simulink model "bhxxx_SL"  (R2016b)
settings: Solver=ode15s  StartTime=0.0  StopTime=60  FixedStep=0.001  RelTol=1e-5  EnableMultiTasking=on
undefined symbols (not defined in the file): b1_damp, b2_damp, b3_damp, b4_damp, g, L1x, L1y, L1z, L2x, L2y, L2z, L3x, L3y, L3z, mass1, mass2, mass3, mass4, Rturn, theta1_0, theta1_dot_0, theta2_0, theta2_dot_0, theta3_0, theta3_dot_0, theta4_0, theta4_dot_0
libraries: simulink x9, discretizing x4, simulink_extras x2
(part 2 of 2)

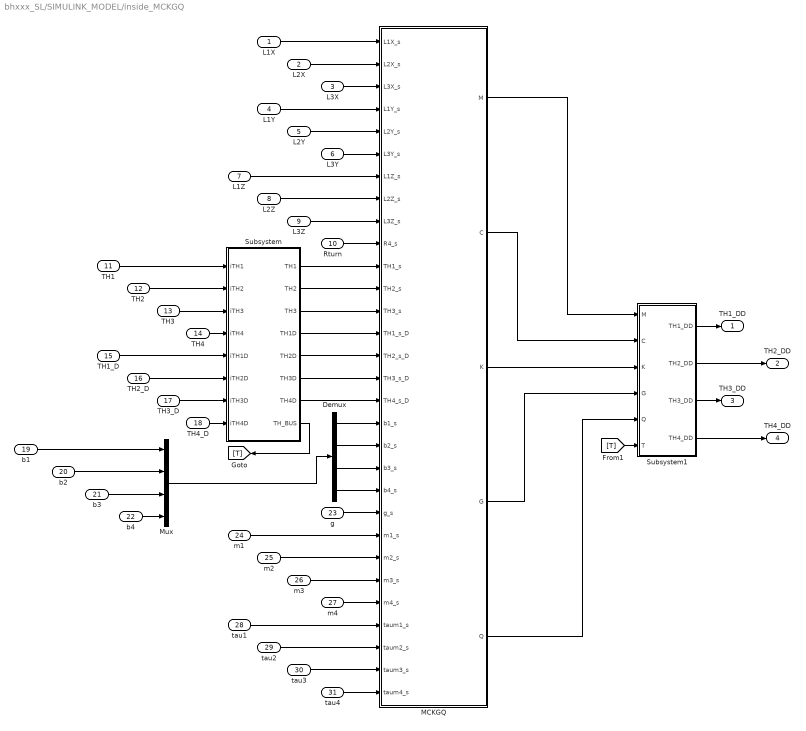
== system bhxxx_SL/SIMULINK_MODEL/inside_MCKGQ ==
  L1X : Inport
  L2X : Inport  Port=2
  L3X : Inport  Port=3
  L1Y : Inport  Port=4
  L2Y : Inport  Port=5
  L3Y : Inport  Port=6
  L1Z : Inport  Port=7
  L2Z : Inport  Port=8
  L3Z : Inport  Port=9
  Rturn : Inport  Port=10
  TH1 : Inport  Port=11
  TH2 : Inport  Port=12
  TH3 : Inport  Port=13
  TH4 : Inport  Port=14
  TH1_D : Inport  Port=15
  TH2_D : Inport  Port=16
  TH3_D : Inport  Port=17
  TH4_D : Inport  Port=18
  b1 : Inport  Port=19
  b2 : Inport  Port=20
  b3 : Inport  Port=21
  b4 : Inport  Port=22
  g : Inport  Port=23
  m1 : Inport  Port=24
  m2 : Inport  Port=25
  m3 : Inport  Port=26
  m4 : Inport  Port=27
  tau1 : Inport  Port=28
  tau2 : Inport  Port=29
  tau3 : Inport  Port=30
  tau4 : Inport  Port=31
  Demux : Demux
  MCKGQ : MATLAB Function  TreatAsAtomicUnit=on
  Mux : Mux
  Subsystem : Subsystem
  Subsystem1 : Subsystem
  TH1_DD : Outport
  TH2_DD : Outport  Port=2
  TH3_DD : Outport  Port=3
  TH4_DD : Outport  Port=4
  wires:
  m2/1 -> MCKGQ/24(m2_s)
  m3/1 -> MCKGQ/25(m3_s)
  m4/1 -> MCKGQ/26(m4_s)
  tau1/1 -> MCKGQ/27(taum1_s)
  g/1 -> MCKGQ/22(g_s)
  m1/1 -> MCKGQ/23(m1_s)
  TH1_D/1 -> Subsystem/5(iTH1D)
  b1/1 -> Mux/1
  b2/1 -> Mux/2
  TH3/1 -> Subsystem/3(iTH3)
  b3/1 -> Mux/3
  TH4_D/1 -> Subsystem/8(iTH4D)
  TH2_D/1 -> Subsystem/6(iTH2D)
  TH3_D/1 -> Subsystem/7(iTH3D)
  b4/1 -> Mux/4
  tau2/1 -> MCKGQ/28(taum2_s)
  tau3/1 -> MCKGQ/29(taum3_s)
  tau4/1 -> MCKGQ/30(taum4_s)
  L2X/1 -> MCKGQ/2(L2X_s)
  L3X/1 -> MCKGQ/3(L3X_s)
  L2Y/1 -> MCKGQ/5(L2Y_s)
  L3Y/1 -> MCKGQ/6(L3Y_s)
  L1Y/1 -> MCKGQ/4(L1Y_s)
  L2Z/1 -> MCKGQ/8(L2Z_s)
  L3Z/1 -> MCKGQ/9(L3Z_s)
  L1Z/1 -> MCKGQ/7(L1Z_s)
  TH1/1 -> Subsystem/1(iTH1)
  Rturn/1 -> MCKGQ/10(R4_s)
  TH2/1 -> Subsystem/2(iTH2)
  L1X/1 -> MCKGQ/1(L1X_s)
  Subsystem/8(TH_BUS) -> [T]
  Subsystem/7(TH4D) -> MCKGQ/17(TH4_s_D)
  Subsystem/6(TH3D) -> MCKGQ/16(TH3_s_D)
  Subsystem/5(TH2D) -> MCKGQ/15(TH2_s_D)
  Subsystem/4(TH1D) -> MCKGQ/14(TH1_s_D)
  Subsystem/3(TH3) -> MCKGQ/13(TH3_s)
  Subsystem/2(TH2) -> MCKGQ/12(TH2_s)
  Subsystem/1(TH1) -> MCKGQ/11(TH1_s)
  TH4/1 -> Subsystem/4(iTH4)
  Demux/1 -> MCKGQ/18(b1_s)
  Demux/2 -> MCKGQ/19(b2_s)
  Demux/3 -> MCKGQ/20(b3_s)
  Demux/4 -> MCKGQ/21(b4_s)
  Mux/1 -> Demux/1
  Subsystem1/1(TH1_DD) -> TH1_DD/1
  Subsystem1/2(TH2_DD) -> TH2_DD/1
  MCKGQ/1(M) -> Subsystem1/1(M)
  MCKGQ/2(C) -> Subsystem1/2(C)
  MCKGQ/3(K) -> Subsystem1/3(K)
  MCKGQ/4(G) -> Subsystem1/4(G)
  MCKGQ/5(Q) -> Subsystem1/5(Q)
  [T] -> Subsystem1/6(T)
  Subsystem1/3(TH3_DD) -> TH3_DD/1
  Subsystem1/4(TH4_DD) -> TH4_DD/1

== system bhxxx_SL/TRAJECTORY/End_Eff_Traj ==
  Bus Creator : BusCreator  Inputs=8
  Demux : Demux  Outputs=3
  Demux1 : Demux  Outputs=3
  From Spreadsheet : FromSpreadsheet  FileName=bh_hello_complete.xlsx  SheetName=COMP_SPLINE _4dof  SampleTime=0.01  ExtrapolationBeforeFirstDataPoint=Hold first value  ExtrapolationAfterLastDataPoint=Hold last value
  Mux : Mux  Inputs=3
  Mux1 : Mux  Inputs=3
  Reshape : Reshape  OutputDimensionality=Column vector (2-D)
  Reshape1 : Reshape  OutputDimensionality=Column vector (2-D)
  EFF_TRAJ : Outport
  wires:
  From Spreadsheet/2 -> Mux/2  "YE"
  From Spreadsheet/3 -> Mux/3  "ZE"
  From Spreadsheet/1 -> Mux/1  "XE"
  From Spreadsheet/4 -> Mux1/1  "DXEDT"
  Bus Creator/1 -> EFF_TRAJ/1
  From Spreadsheet/6 -> Mux1/3  "DZEDT"
  From Spreadsheet/5 -> Mux1/2  "DYEDT"
  Demux/1 -> Bus Creator/6  "DXEDT"
  Demux/2 -> Bus Creator/7  "DYEDT"
  Demux/3 -> Bus Creator/8  "DZEDT"
  Demux1/1 -> Bus Creator/1  "XE"
  Demux1/2 -> Bus Creator/2  "YE"
  Demux1/3 -> Bus Creator/3  "ZE"
  Mux/1 -> Reshape/1  "XYZ"
  Mux1/1 -> Reshape1/1
  Reshape/1 -> Bus Creator/4, Demux1/1  "XYZ_POS"
  Reshape1/1 -> Demux/1, Bus Creator/5  "XYZ_VEL"

== system bhxxx_SL/TRAJECTORY/Subsystem ==
  In1 : Inport
  In2 : Inport  Port=2
  Mux2 : Mux  Inputs=2
  Reshape : Reshape  OutputDimensionality=Column vector (2-D)
  Reshape1 : Reshape  OutputDimensionality=Column vector (2-D)
  Selector : Selector  InputPortWidth=8  IndexOptions=Index vector (dialog)  Indices=[1 5]  OutputSizes=1
  Selector1 : Selector  InputPortWidth=8  IndexOptions=Index vector (dialog)  Indices=[2 6]  OutputSizes=1
  Selector2 : Selector  InputPortWidth=8  IndexOptions=Index vector (dialog)  Indices=[3 7]  OutputSizes=1
  Selector3 : Selector  InputPortWidth=8  IndexOptions=Index vector (dialog)  Indices=[4 8]  OutputSizes=1
  Out1 : Outport
  Out2 : Outport  Port=2
  Out3 : Outport  Port=3
  Out4 : Outport  Port=4
  wires:
  In1/1 -> Reshape/1
  In2/1 -> Reshape1/1
  Reshape/1 -> Mux2/1
  Reshape1/1 -> Mux2/2
  Selector2/1 -> Out3/1
  Selector1/1 -> Out2/1
  Selector/1 -> Out1/1
  Mux2/1 -> Selector1/1, Selector/1, Selector2/1, Selector3/1
  Selector3/1 -> Out4/1

== system bhxxx_SL/TRAJECTORY/XY_compare ==
  XY_GOAL : Inport
  XY : Inport  Port=2
  Bus Selector1 : BusSelector  OutputSignals=XE,YE,ZE
  Demux : Demux  Outputs=3
  Mux : Mux  Inputs=2
  Mux1 : Mux  Inputs=2
  Mux2 : Mux  Inputs=2
  X : Outport
  Y : Outport  Port=2
  Z : Outport  Port=3
  wires:
  XY_GOAL/1 -> Bus Selector1/1
  XY/1 -> Demux/1
  Bus Selector1/1 -> Mux/1  "<XE>"
  Demux/1 -> Mux/2
  Bus Selector1/2 -> Mux1/1  "<YE>"
  Demux/2 -> Mux1/2
  Mux/1 -> X/1
  Mux1/1 -> Y/1
  Mux2/1 -> Z/1
  Bus Selector1/3 -> Mux2/1  "<ZE>"
  Demux/3 -> Mux2/2

== system bhxxx_SL/TRAJECTORY/get_XYDOT ==
  In1 : Inport
  Bus Selector2 : BusSelector  OutputSignals=DXEDT,DYEDT,DZEDT
  Mux2 : Mux  Inputs=3
  Reshape : Reshape  OutputDimensionality=Column vector (2-D)
  Out1 : Outport
  wires:
  Bus Selector2/1 -> Mux2/1  "<DXEDT>"
  Bus Selector2/2 -> Mux2/2  "<DYEDT>"
  In1/1 -> Bus Selector2/1
  Mux2/1 -> Reshape/1
  Reshape/1 -> Out1/1  "XY_DOT"
  Bus Selector2/3 -> Mux2/3  "<DZEDT>"

== system bhxxx_SL/VIEW/XYZ_EFF_COMPARE ==
  CMD_BUS : Inport
  PLANT_BUS : Inport  Port=2
  Bus Selector1 : BusSelector  OutputSignals=CALC_POS_BUS.WF_pos_EFF
  Bus Selector4 : BusSelector  OutputSignals=XYZ_BUS.XYZ_POS
  Mux : Mux  Inputs=2
  Reshape1 : Reshape  OutputDimensionality=Column vector (2-D)
  Reshape2 : Reshape  OutputDimensionality=Column vector (2-D)
  Selector : Selector  InputPortWidth=6  IndexOptions=Index vector (dialog)  Indices=[1 4]  OutputSizes=1
  Selector1 : Selector  InputPortWidth=6  IndexOptions=Index vector (dialog)  Indices=[2 5]  OutputSizes=1
  Selector2 : Selector  InputPortWidth=6  IndexOptions=Index vector (dialog)  Indices=[3 6]  OutputSizes=1
  X : Outport
  Y : Outport  Port=2
  Z : Outport  Port=3
  wires:
  CMD_BUS/1 -> Bus Selector4/1
  PLANT_BUS/1 -> Bus Selector1/1
  Bus Selector4/1 -> Reshape1/1  "<XYZ_POS>"
  Bus Selector1/1 -> Reshape2/1  "<WF_pos_EFF>"
  Reshape1/1 -> Mux/1
  Reshape2/1 -> Mux/2
  Mux/1 -> Selector2/1, Selector1/1, Selector/1
  Selector2/1 -> Z/1
  Selector1/1 -> Y/1
  Selector/1 -> X/1

== system bhxxx_SL/Create_PLANT_BUS/Subsystem1/Subsystem1 ==
  mg_signed : Inport
  Constant : Constant  Value=0
  Mux : Mux  Inputs=3
  Reshape : Reshape  OutputDimensionality=Column vector (2-D)
  COL : Outport
  wires:
  mg_signed/1 -> Mux/3
  Constant/1 -> Mux/2, Mux/1
  Mux/1 -> Reshape/1
  Reshape/1 -> COL/1

== system bhxxx_SL/Create_PLANT_BUS/Subsystem1/Subsystem2 ==
  mg_signed : Inport
  Constant : Constant  Value=0
  Mux : Mux  Inputs=3
  Reshape : Reshape  OutputDimensionality=Column vector (2-D)
  COL : Outport
  wires:
  mg_signed/1 -> Mux/3
  Constant/1 -> Mux/2, Mux/1
  Mux/1 -> Reshape/1
  Reshape/1 -> COL/1

== system bhxxx_SL/Create_PLANT_BUS/Subsystem1/Subsystem3 ==
  mg_signed : Inport
  Constant : Constant  Value=0
  Mux : Mux  Inputs=3
  Reshape : Reshape  OutputDimensionality=Column vector (2-D)
  COL : Outport
  wires:
  mg_signed/1 -> Mux/3
  Constant/1 -> Mux/2, Mux/1
  Mux/1 -> Reshape/1
  Reshape/1 -> COL/1

== system bhxxx_SL/Create_PLANT_BUS/Subsystem1/Subsystem4 ==
  mg_signed : Inport
  Constant : Constant  Value=0
  Mux : Mux  Inputs=3
  Reshape : Reshape  OutputDimensionality=Column vector (2-D)
  COL : Outport
  wires:
  mg_signed/1 -> Mux/3
  Constant/1 -> Mux/2, Mux/1
  Mux/1 -> Reshape/1
  Reshape/1 -> COL/1

== system bhxxx_SL/Create_PLANT_BUS/Subsystem1/Subsystem5 ==
  mg_signed : Inport
  Constant : Constant  Value=0
  Mux : Mux  Inputs=3
  Reshape : Reshape  OutputDimensionality=Column vector (2-D)
  COL : Outport
  wires:
  mg_signed/1 -> Mux/3
  Constant/1 -> Mux/2, Mux/1
  Mux/1 -> Reshape/1
  Reshape/1 -> COL/1

== system bhxxx_SL/Create_PLANT_BUS/Subsystem1/Subsystem6 ==
  mg_signed : Inport
  Constant : Constant  Value=0
  Mux : Mux  Inputs=3
  Reshape : Reshape  OutputDimensionality=Column vector (2-D)
  COL : Outport
  wires:
  mg_signed/1 -> Mux/3
  Constant/1 -> Mux/2, Mux/1
  Mux/1 -> Reshape/1
  Reshape/1 -> COL/1

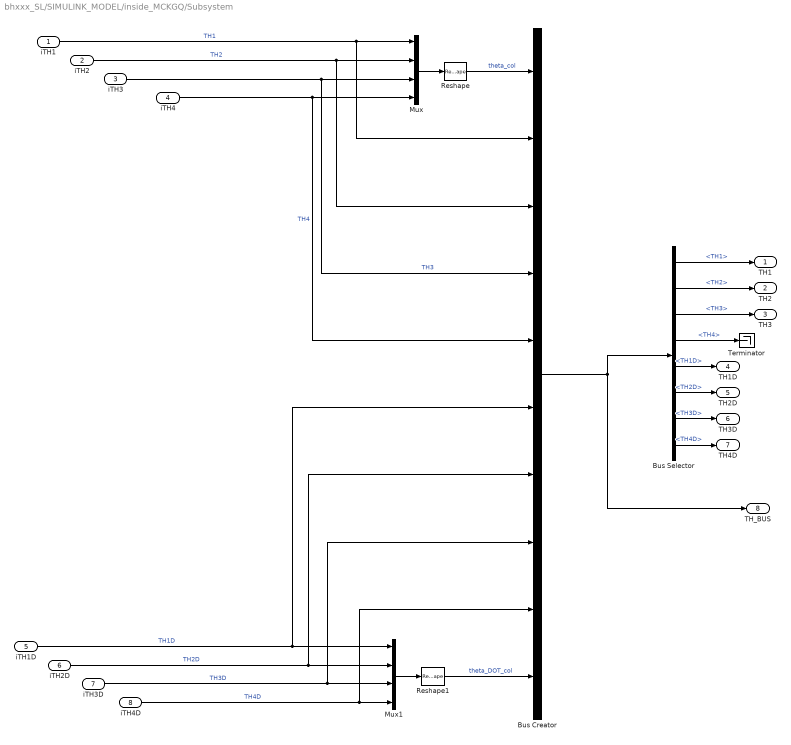
== system bhxxx_SL/SIMULINK_MODEL/inside_MCKGQ/Subsystem ==
  iTH1 : Inport
  iTH2 : Inport  Port=2
  iTH3 : Inport  Port=3
  iTH4 : Inport  Port=4
  iTH1D : Inport  Port=5
  iTH2D : Inport  Port=6
  iTH3D : Inport  Port=7
  iTH4D : Inport  Port=8
  Bus Creator : BusCreator  Inputs=10
  Bus Selector : BusSelector  OutputSignals=TH1,TH2,TH3,TH4,TH1D,TH2D,TH3D,TH4D
  Mux : Mux
  Mux1 : Mux
  Reshape : Reshape  OutputDimensionality=Column vector (2-D)
  Reshape1 : Reshape  OutputDimensionality=Column vector (2-D)
  Terminator : Terminator
  TH1 : Outport
  TH2 : Outport  Port=2
  TH3 : Outport  Port=3
  TH1D : Outport  Port=4
  TH2D : Outport  Port=5
  TH3D : Outport  Port=6
  TH4D : Outport  Port=7
  TH_BUS : Outport  Port=8
  wires:
  iTH2/1 -> Bus Creator/3, Mux/2  "TH2"
  iTH1/1 -> Bus Creator/2, Mux/1  "TH1"
  iTH2D/1 -> Bus Creator/7, Mux1/2  "TH2D"
  iTH1D/1 -> Bus Creator/6, Mux1/1  "TH1D"
  Mux/1 -> Reshape/1
  Mux1/1 -> Reshape1/1
  Reshape/1 -> Bus Creator/1  "theta_col"
  Reshape1/1 -> Bus Creator/10  "theta_DOT_col"
  Bus Creator/1 -> TH_BUS/1, Bus Selector/1
  iTH3D/1 -> Bus Creator/8, Mux1/3  "TH3D"
  iTH3/1 -> Bus Creator/4, Mux/3  "TH3"
  Bus Selector/1 -> TH1/1  "<TH1>"
  Bus Selector/2 -> TH2/1  "<TH2>"
  Bus Selector/3 -> TH3/1  "<TH3>"
  Bus Selector/5 -> TH1D/1  "<TH1D>"
  Bus Selector/6 -> TH2D/1  "<TH2D>"
  Bus Selector/7 -> TH3D/1  "<TH3D>"
  iTH4/1 -> Bus Creator/5, Mux/4  "TH4"
  iTH4D/1 -> Bus Creator/9, Mux1/4  "TH4D"
  Bus Selector/4 -> Terminator/1  "<TH4>"
  Bus Selector/8 -> TH4D/1  "<TH4D>"

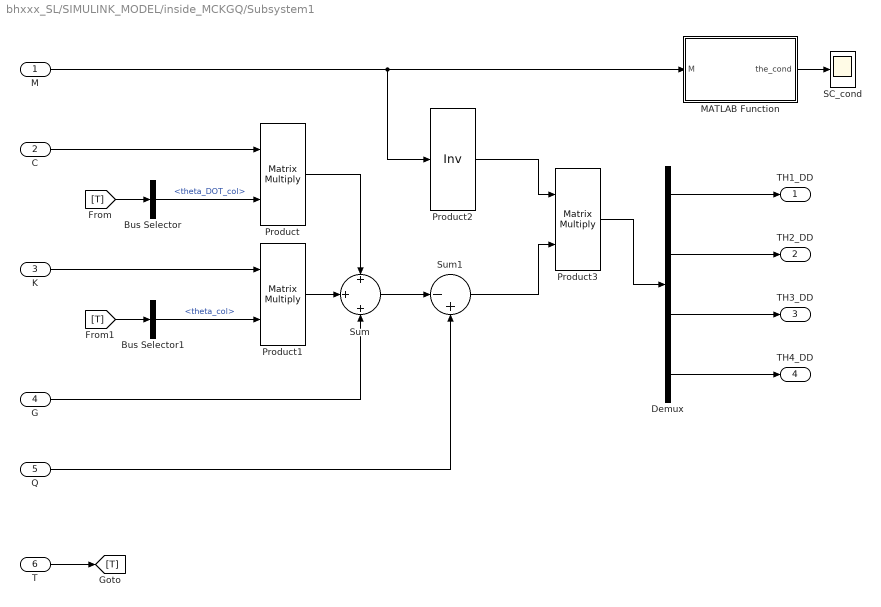
== system bhxxx_SL/SIMULINK_MODEL/inside_MCKGQ/Subsystem1 ==
  M : Inport
  C : Inport  Port=2
  K : Inport  Port=3
  G : Inport  Port=4
  Q : Inport  Port=5
  T : Inport  Port=6
  Bus Selector : BusSelector  OutputSignals=theta_DOT_col
  Bus Selector1 : BusSelector  OutputSignals=theta_col
  Demux : Demux
  MATLAB Function : MATLAB Function  TreatAsAtomicUnit=on
  Product : Product  Multiplication=Matrix(*)
  Product1 : Product  Multiplication=Matrix(*)
  Product2 : Product  Inputs=/  Multiplication=Matrix(*)
  Product3 : Product  Multiplication=Matrix(*)
  SC_cond : Scope
  Sum : Sum  Inputs=+|+|+
  Sum1 : Sum  Inputs=|-+
  TH1_DD : Outport
  TH2_DD : Outport  Port=2
  TH3_DD : Outport  Port=3
  TH4_DD : Outport  Port=4
  wires:
  T/1 -> [T]
  C/1 -> Product/1
  [T] -> Bus Selector/1
  Bus Selector/1 -> Product/2  "<theta_DOT_col>"
  K/1 -> Product1/1
  [T] -> Bus Selector1/1
  Bus Selector1/1 -> Product1/2  "<theta_col>"
  Q/1 -> Sum1/2
  Product1/1 -> Sum/2
  G/1 -> Sum/3
  Product/1 -> Sum/1
  Sum/1 -> Sum1/1
  M/1 -> Product2/1, MATLAB Function/1(M)
  Product2/1 -> Product3/1
  Sum1/1 -> Product3/2
  Product3/1 -> Demux/1
  Demux/1 -> TH1_DD/1
  Demux/2 -> TH2_DD/1
  MATLAB Function/1(the_cond) -> SC_cond/1
  Demux/3 -> TH3_DD/1
  Demux/4 -> TH4_DD/1

== matlab function bhxxx_SL/TRAJECTORY/THE_J ==
  data: L1Y_s input; the_J output; L2Y_s input; L3Y_s input; theta1 input; theta2 input; theta3 input; theta4 input
function the_J = THE_J(L1Y_s,L2Y_s,L3Y_s,theta1,theta2,theta3,theta4)
%#codegen

%    This function was generated by the Symbolic Math Toolbox version 7.0.
%    13-Sep-2016 14:49:06

the_J = reshape([sin(theta4).*(L2Y_s.*sin(theta1+theta2)+L1Y_s.*sin(theta1)+L3Y_s.*sin(theta1+theta2+theta3)),-cos(theta4).*(L2Y_s.*sin(theta1+theta2)+L1Y_s.*sin(theta1)+L3Y_s.*sin(theta1+theta2+theta3)),L2Y_s.*cos(theta1+theta2)+L1Y_s.*cos(theta1)+L3Y_s.*cos(theta1+theta2+theta3),sin(theta4).*(L2Y_s.*sin(theta1+theta2)+L3Y_s.*sin(theta1+theta2+theta3)),-cos(theta4).*(L2Y_s.*sin(theta1+theta2)+L3Y_s.*sin(theta1+theta2+theta3)),L2Y_s.*cos(theta1+theta2)+L3Y_s.*cos(theta1+theta2+theta3),L3Y_s.*sin(theta1+theta2+theta3).*sin(theta4),-L3Y_s.*sin(theta1+theta2+theta3).*cos(theta4),L3Y_s.*cos(theta1+theta2+theta3),-cos(theta4).*(L2Y_s.*cos(theta1+theta2)+L1Y_s.*cos(theta1)+L3Y_s.*cos(theta1+theta2+theta3)),-sin(theta4).*(L2Y_s.*cos(theta1+theta2)+L1Y_s.*cos(theta1)+L3Y_s.*cos(theta1+theta2+theta3)),0.0],[3,4]);

== matlab function bhxxx_SL/SIMULINK_MODEL/inside_MCKGQ/MCKGQ ==
  data: L1X_s input; M output; L2X_s input; L3X_s input; L1Y_s input; L2Y_s input; L3Y_s input; L1Z_s input; L2Z_s input; L3Z_s input; R4_s input; TH1_s input; TH2_s input; TH3_s input; TH1_s_D input; TH2_s_D input; TH3_s_D input; TH4_s_D input; b1_s input; b2_s input; b3_s input; b4_s input; g_s input; m1_s input; m2_s input; m3_s input; m4_s input; taum1_s input; taum2_s input; taum3_s input; taum4_s input; C output; K output; G output; Q output
function [M,C,K,G,Q] = MCKGQ(L1X_s,L2X_s,L3X_s,L1Y_s,L2Y_s,L3Y_s,L1Z_s,L2Z_s,L3Z_s,R4_s,TH1_s,TH2_s,TH3_s,TH1_s_D,TH2_s_D,TH3_s_D,TH4_s_D,b1_s,b2_s,b3_s,b4_s,g_s,m1_s,m2_s,m3_s,m4_s,taum1_s,taum2_s,taum3_s,taum4_s)
%#codegen

%    This function was generated by the Symbolic Math Toolbox version 7.0.
%    13-Sep-2016 13:01:16

M = reshape([L1Y_s.^2.*m1_s.*(1.0./3.0)+L1Y_s.^2.*m2_s+L1Y_s.^2.*m3_s+L2Y_s.^2.*m2_s.*(1.0./3.0)+L2Y_s.^2.*m3_s+L3Y_s.^2.*m3_s.*(1.0./3.0)+L1Z_s.^2.*m1_s.*(1.0./1.2e1)+L2Z_s.^2.*m2_s.*(1.0./1.2e1)+L3Z_s.^2.*m3_s.*(1.0./1.2e1)+L1Y_s.*L2Y_s.*m2_s.*cos(TH2_s)+L1Y_s.*L2Y_s.*m3_s.*cos(TH2_s).*2.0+L2Y_s.*L3Y_s.*m3_s.*cos(TH3_s)+L1Y_s.*L3Y_s.*m3_s.*cos(TH2_s+TH3_s),L2Y_s.^2.*m2_s.*(1.0./3.0)+L2Y_s.^2.*m3_s+L3Y_s.^2.*m3_s.*(1.0./3.0)+L2Z_s.^2.*m2_s.*(1.0./1.2e1)+L3Z_s.^2.*m3_s.*(1.0./1.2e1)+L1Y_s.*L2Y_s.*m2_s.*cos(TH2_s).*(1.0./2.0)+L1Y_s.*L2Y_s.*m3_s.*cos(TH2_s)+L2Y_s.*L3Y_s.*m3_s.*cos(TH3_s)+L1Y_s.*L3Y_s.*m3_s.*cos(TH2_s+TH3_s).*(1.0./2.0),m3_s.*(L3Y_s.^2.*4.0+L3Z_s.^2+L1Y_s.*L3Y_s.*cos(TH2_s+TH3_s).*6.0+L2Y_s.*L3Y_s.*cos(TH3_s).*6.0).*(1.0./1.2e1),0.0,L2Y_s.^2.*m2_s.*(1.0./3.0)+L2Y_s.^2.*m3_s+L3Y_s.^2.*m3_s.*(1.0./3.0)+L2Z_s.^2.*m2_s.*(1.0./1.2e1)+L3Z_s.^2.*m3_s.*(1.0./1.2e1)+L1Y_s.*L2Y_s.*m2_s.*cos(TH2_s).*(1.0./2.0)+L1Y_s.*L2Y_s.*m3_s.*cos(TH2_s)+L2Y_s.*L3Y_s.*m3_s.*cos(TH3_s)+L1Y_s.*L3Y_s.*m3_s.*cos(TH2_s+TH3_s).*(1.0./2.0),L2Y_s.^2.*m2_s.*(1.0./3.0)+L2Y_s.^2.*m3_s+L3Y_s.^2.*m3_s.*(1.0./3.0)+L2Z_s.^2.*m2_s.*(1.0./1.2e1)+L3Z_s.^2.*m3_s.*(1.0./1.2e1)+L2Y_s.*L3Y_s.*m3_s.*cos(TH3_s),m3_s.*(L3Y_s.^2.*4.0+L3Z_s.^2+L2Y_s.*L3Y_s.*cos(TH3_s).*6.0).*(1.0./1.2e1),0.0,m3_s.*(L3Y_s.^2.*4.0+L3Z_s.^2+L1Y_s.*L3Y_s.*cos(TH2_s+TH3_s).*6.0+L2Y_s.*L3Y_s.*cos(TH3_s).*6.0).*(1.0./1.2e1),m3_s.*(L3Y_s.^2.*4.0+L3Z_s.^2+L2Y_s.*L3Y_s.*cos(TH3_s).*6.0).*(1.0./1.2e1),m3_s.*(L3Y_s.^2.*4.0+L3Z_s.^2).*(1.0./1.2e1),0.0,0.0,0.0,0.0,L1X_s.^2.*m1_s.*(1.0./1.2e1)+L2X_s.^2.*m2_s.*(1.0./1.2e1)+L3X_s.^2.*m3_s.*(1.0./1.2e1)+L1Y_s.^2.*m1_s.*(1.0./6.0)+L1Y_s.^2.*m2_s.*(1.0./2.0)+L1Y_s.^2.*m3_s.*(1.0./2.0)+L2Y_s.^2.*m2_s.*(1.0./6.0)+L2Y_s.^2.*m3_s.*(1.0./2.0)+L3Y_s.^2.*m3_s.*(1.0./6.0)+L1Z_s.^2.*m1_s.*(1.0./2.4e1)+L2Z_s.^2.*m2_s.*(1.0./2.4e1)+L3Z_s.^2.*m3_s.*(1.0./2.4e1)+R4_s.^2.*m4_s.*(1.0./2.0)+L3Y_s.^2.*m3_s.*cos(TH1_s.*2.0+TH2_s.*2.0+TH3_s.*2.0).*(1.0./6.0)-L3Z_s.^2.*m3_s.*cos(TH1_s.*2.0+TH2_s.*2.0+TH3_s.*2.0).*(1.0./2.4e1)+L1Y_s.^2.*m1_s.*cos(TH1_s.*2.0).*(1.0./6.0)+L1Y_s.^2.*m2_s.*cos(TH1_s.*2.0).*(1.0./2.0)+L1Y_s.^2.*m3_s.*cos(TH1_s.*2.0).*(1.0./2.0)-L1Z_s.^2.*m1_s.*cos(TH1_s.*2.0).*(1.0./2.4e1)+L2Y_s.^2.*m2_s.*cos(TH1_s.*2.0+TH2_s.*2.0).*(1.0./6.0)+L2Y_s.^2.*m3_s.*cos(TH1_s.*2.0+TH2_s.*2.0).*(1.0./2.0)-L2Z_s.^2.*m2_s.*cos(TH1_s.*2.0+TH2_s.*2.0).*(1.0./2.4e1)+L1Y_s.*L2Y_s.*m2_s.*cos(TH2_s).*(1.0./2.0)+L1Y_s.*L2Y_s.*m3_s.*cos(TH2_s)+L2Y_s.*L3Y_s.*m3_s.*cos(TH3_s).*(1.0./2.0)+L1Y_s.*L2Y_s.*m2_s.*cos(TH1_s.*2.0+TH2_s).*(1.0./2.0)+L1Y_s.*L2Y_s.*m3_s.*cos(TH1_s.*2.0+TH2_s)+L1Y_s.*L3Y_s.*m3_s.*cos(TH1_s.*2.0+TH2_s+TH3_s).*(1.0./2.0)+L1Y_s.*L3Y_s.*m3_s.*cos(TH2_s+TH3_s).*(1.0./2.0)+L2Y_s.*L3Y_s.*m3_s.*cos(TH1_s.*2.0+TH2_s.*2.0+TH3_s).*(1.0./2.0)],[4,4]);
if nargout > 1
    C = reshape([-L1Y_s.*L3Y_s.*TH2_s_D.*m3_s.*sin(TH2_s+TH3_s)-L1Y_s.*L3Y_s.*TH3_s_D.*m3_s.*sin(TH2_s+TH3_s)-L1Y_s.*L2Y_s.*TH2_s_D.*m2_s.*sin(TH2_s)-L1Y_s.*L2Y_s.*TH2_s_D.*m3_s.*sin(TH2_s).*2.0-L2Y_s.*L3Y_s.*TH3_s_D.*m3_s.*sin(TH3_s),L1Y_s.*L3Y_s.*TH1_s_D.*m3_s.*sin(TH2_s+TH3_s).*(1.0./2.0)+L1Y_s.*L2Y_s.*TH1_s_D.*m2_s.*sin(TH2_s).*(1.0./2.0)+L1Y_s.*L2Y_s.*TH1_s_D.*m3_s.*sin(TH2_s)-L2Y_s.*L3Y_s.*TH3_s_D.*m3_s.*sin(TH3_s),L3Y_s.*m3_s.*(L1Y_s.*TH1_s_D.*sin(TH2_s+TH3_s)+L2Y_s.*TH1_s_D.*sin(TH3_s)+L2Y_s.*TH2_s_D.*sin(TH3_s).*2.0).*(1.0./2.0),TH4_s_D.*(L3Y_s.^2.*m3_s.*sin(TH1_s.*2.0+TH2_s.*2.0+TH3_s.*2.0).*4.0-L3Z_s.^2.*m3_s.*sin(TH1_s.*2.0+TH2_s.*2.0+TH3_s.*2.0)+L1Y_s.^2.*m1_s.*sin(TH1_s.*2.0).*4.0+L1Y_s.^2.*m2_s.*sin(TH1_s.*2.0).*1.2e1+L1Y_s.^2.*m3_s.*sin(TH1_s.*2.0).*1.2e1-L1Z_s.^2.*m1_s.*sin(TH1_s.*2.0)+L2Y_s.^2.*m2_s.*sin(TH1_s.*2.0+TH2_s.*2.0).*4.0+L2Y_s.^2.*m3_s.*sin(TH1_s.*2.0+TH2_s.*2.0).*1.2e1-L2Z_s.^2.*m2_s.*sin(TH1_s.*2.0+TH2_s.*2.0)+L1Y_s.*L2Y_s.*m2_s.*sin(TH1_s.*2.0+TH2_s).*1.2e1+L1Y_s.*L2Y_s.*m3_s.*sin(TH1_s.*2.0+TH2_s).*2.4e1+L1Y_s.*L3Y_s.*m3_s.*sin(TH1_s.*2.0+TH2_s+TH3_s).*1.2e1+L2Y_s.*L3Y_s.*m3_s.*sin(TH1_s.*2.0+TH2_s.*2.0+TH3_s).*1.2e1).*(-1.0./1.2e1),L1Y_s.*L3Y_s.*TH2_s_D.*m3_s.*sin(TH2_s+TH3_s).*(-1.0./2.0)-L1Y_s.*L3Y_s.*TH3_s_D.*m3_s.*sin(TH2_s+TH3_s)-L1Y_s.*L2Y_s.*TH2_s_D.*m2_s.*sin(TH2_s).*(1.0./2.0)-L1Y_s.*L2Y_s.*TH2_s_D.*m3_s.*sin(TH2_s)-L2Y_s.*L3Y_s.*TH3_s_D.*m3_s.*sin(TH3_s),-L2Y_s.*L3Y_s.*TH3_s_D.*m3_s.*sin(TH3_s),L2Y_s.*L3Y_s.*TH2_s_D.*m3_s.*sin(TH3_s).*(1.0./2.0),TH4_s_D.*(L3Y_s.^2.*m3_s.*sin(TH1_s.*2.0+TH2_s.*2.0+TH3_s.*2.0).*4.0-L3Z_s.^2.*m3_s.*sin(TH1_s.*2.0+TH2_s.*2.0+TH3_s.*2.0)+L2Y_s.^2.*m2_s.*sin(TH1_s.*2.0+TH2_s.*2.0).*4.0+L2Y_s.^2.*m3_s.*sin(TH1_s.*2.0+TH2_s.*2.0).*1.2e1-L2Z_s.^2.*m2_s.*sin(TH1_s.*2.0+TH2_s.*2.0)+L1Y_s.*L2Y_s.*m2_s.*sin(TH2_s).*6.0+L1Y_s.*L2Y_s.*m3_s.*sin(TH2_s).*1.2e1+L1Y_s.*L2Y_s.*m2_s.*sin(TH1_s.*2.0+TH2_s).*6.0+L1Y_s.*L2Y_s.*m3_s.*sin(TH1_s.*2.0+TH2_s).*1.2e1+L1Y_s.*L3Y_s.*m3_s.*sin(TH1_s.*2.0+TH2_s+TH3_s).*6.0+L1Y_s.*L3Y_s.*m3_s.*sin(TH2_s+TH3_s).*6.0+L2Y_s.*L3Y_s.*m3_s.*sin(TH1_s.*2.0+TH2_s.*2.0+TH3_s).*1.2e1).*(-1.0./1.2e1),L3Y_s.*TH3_s_D.*m3_s.*(L1Y_s.*sin(TH2_s+TH3_s)+L2Y_s.*sin(TH3_s)).*(-1.0./2.0),L2Y_s.*L3Y_s.*TH3_s_D.*m3_s.*sin(TH3_s).*(-1.0./2.0),0.0,TH4_s_D.*m3_s.*(L3Y_s.^2.*sin(TH1_s.*2.0+TH2_s.*2.0+TH3_s.*2.0).*4.0-L3Z_s.^2.*sin(TH1_s.*2.0+TH2_s.*2.0+TH3_s.*2.0)+L1Y_s.*L3Y_s.*sin(TH1_s.*2.0+TH2_s+TH3_s).*6.0+L1Y_s.*L3Y_s.*sin(TH2_s+TH3_s).*6.0+L2Y_s.*L3Y_s.*sin(TH1_s.*2.0+TH2_s.*2.0+TH3_s).*6.0+L2Y_s.*L3Y_s.*sin(TH3_s).*6.0).*(-1.0./1.2e1),TH4_s_D.*(L3Y_s.^2.*m3_s.*sin(TH1_s.*2.0+TH2_s.*2.0+TH3_s.*2.0).*4.0-L3Z_s.^2.*m3_s.*sin(TH1_s.*2.0+TH2_s.*2.0+TH3_s.*2.0)+L1Y_s.^2.*m1_s.*sin(TH1_s.*2.0).*4.0+L1Y_s.^2.*m2_s.*sin(TH1_s.*2.0).*1.2e1+L1Y_s.^2.*m3_s.*sin(TH1_s.*2.0).*1.2e1-L1Z_s.^2.*m1_s.*sin(TH1_s.*2.0)+L2Y_s.^2.*m2_s.*sin(TH1_s.*2.0+TH2_s.*2.0).*4.0+L2Y_s.^2.*m3_s.*sin(TH1_s.*2.0+TH2_s.*2.0).*1.2e1-L2Z_s.^2.*m2_s.*sin(TH1_s.*2.0+TH2_s.*2.0)+L1Y_s.*L2Y_s.*m2_s.*sin(TH1_s.*2.0+TH2_s).*1.2e1+L1Y_s.*L2Y_s.*m3_s.*sin(TH1_s.*2.0+TH2_s).*2.4e1+L1Y_s.*L3Y_s.*m3_s.*sin(TH1_s.*2.0+TH2_s+TH3_s).*1.2e1+L2Y_s.*L3Y_s.*m3_s.*sin(TH1_s.*2.0+TH2_s.*2.0+TH3_s).*1.2e1).*(1.0./2.4e1),TH4_s_D.*(L3Y_s.^2.*m3_s.*sin(TH1_s.*2.0+TH2_s.*2.0+TH3_s.*2.0).*4.0-L3Z_s.^2.*m3_s.*sin(TH1_s.*2.0+TH2_s.*2.0+TH3_s.*2.0)+L2Y_s.^2.*m2_s.*sin(TH1_s.*2.0+TH2_s.*2.0).*4.0+L2Y_s.^2.*m3_s.*sin(TH1_s.*2.0+TH2_s.*2.0).*1.2e1-L2Z_s.^2.*m2_s.*sin(TH1_s.*2.0+TH2_s.*2.0)+L1Y_s.*L2Y_s.*m2_s.*sin(TH2_s).*6.0+L1Y_s.*L2Y_s.*m3_s.*sin(TH2_s).*1.2e1+L1Y_s.*L2Y_s.*m2_s.*sin(TH1_s.*2.0+TH2_s).*6.0+L1Y_s.*L2Y_s.*m3_s.*sin(TH1_s.*2.0+TH2_s).*1.2e1+L1Y_s.*L3Y_s.*m3_s.*sin(TH1_s.*2.0+TH2_s+TH3_s).*6.0+L1Y_s.*L3Y_s.*m3_s.*sin(TH2_s+TH3_s).*6.0+L2Y_s.*L3Y_s.*m3_s.*sin(TH1_s.*2.0+TH2_s.*2.0+TH3_s).*1.2e1).*(1.0./2.4e1),TH4_s_D.*m3_s.*(L3Y_s.^2.*sin(TH1_s.*2.0+TH2_s.*2.0+TH3_s.*2.0).*4.0-L3Z_s.^2.*sin(TH1_s.*2.0+TH2_s.*2.0+TH3_s.*2.0)+L1Y_s.*L3Y_s.*sin(TH1_s.*2.0+TH2_s+TH3_s).*6.0+L1Y_s.*L3Y_s.*sin(TH2_s+TH3_s).*6.0+L2Y_s.*L3Y_s.*sin(TH1_s.*2.0+TH2_s.*2.0+TH3_s).*6.0+L2Y_s.*L3Y_s.*sin(TH3_s).*6.0).*(1.0./2.4e1),0.0],[4,4]);
end
if nargout > 2
    K = reshape([0.0,0.0,0.0,0.0,0.0,0.0,0.0,0.0,0.0,0.0,0.0,0.0,0.0,0.0,0.0,0.0],[4,4]);
end
if nargout > 3
    G = [g_s.*(L2Y_s.*m2_s.*cos(TH1_s+TH2_s)+L2Y_s.*m3_s.*cos(TH1_s+TH2_s).*2.0+L1Y_s.*m1_s.*cos(TH1_s)+L1Y_s.*m2_s.*cos(TH1_s).*2.0+L1Y_s.*m3_s.*cos(TH1_s).*2.0+L3Y_s.*m3_s.*cos(TH1_s+TH2_s+TH3_s)).*(1.0./2.0);L3Y_s.*g_s.*m3_s.*cos(TH1_s+TH2_s+TH3_s).*(1.0./2.0)+L2Y_s.*g_s.*m2_s.*cos(TH1_s+TH2_s).*(1.0./2.0)+L2Y_s.*g_s.*m3_s.*cos(TH1_s+TH2_s);L3Y_s.*g_s.*m3_s.*cos(TH1_s+TH2_s+TH3_s).*(1.0./2.0);0.0];
end
if nargout > 4
    Q = [taum1_s-TH1_s_D.*b1_s;taum2_s-TH2_s_D.*b2_s;taum3_s-TH3_s_D.*b3_s;taum4_s-TH4_s_D.*b4_s];
end

== matlab function bhxxx_SL/TRAJECTORY/CALC_THETA_DOT ==
  data: J input; TH_DOT output; XY_DOT input; lambda_sq input; alt_TH_DOT output
function [TH_DOT, alt_TH_DOT] = calc_TH_DOT(J, XY_DOT, lambda_sq)
%#codegen

    %% so our problem is this:
    %     J*q_dot = x_dot
    %
    % so a solution is:
    %
    %      q_dot = pinv(J) * x_dot
    
    TH_DOT = pinv(J) * XY_DOT;

    %% we can also penalise the q_dot by applying a weight to it.
    %  this will give us a solution where we get a "smaller" q_dot.  This
    %  acts as a "dampening" agent ... and we notice it most at startup.
    
    % consider solving the REGULARISED problem
    %     [       J_mxn  ] * q_dot =  [ x_dot ]
    %     [lamb^2*I_nxn  ]            [ 0_nx1 ]
    %
    % which we'll wite as:
    %
    %              new_A * q_dot = new_b
    %
    % so a solution is:
    %
    %      q_dot = pinv(new_A) * new_b
    
    [m, n]     = size(J); 
    I_mat      = eye( n ); 
    new_A      = [ J;
                   lambda_sq * I_mat];

    new_b      = [ XY_DOT;
                   zeros(n,1) ];

    alt_TH_DOT = pinv( new_A  ) * new_b;
end

== matlab function bhxxx_SL/SIMULINK_MODEL/inside_MCKGQ/Subsystem1/MATLAB Function ==
  data: M input; the_cond output
function the_cond = COND(M)
%#codegen

the_cond = cond(M);

end

== matlab function bhxxx_SL/TRAJECTORY/THE_XEYE ==
  data: L1Y_s input; XE output; L2Y_s input; L3Y_s input; theta1 input; theta2 input; theta3 input; theta4 input; YE output; ZE output
function [XE,YE,ZE] = THE_XEYE(L1Y_s,L2Y_s,L3Y_s,theta1,theta2,theta3,theta4)
%#codegen

%    This function was generated by the Symbolic Math Toolbox version 7.0.
%    13-Sep-2016 15:29:58

XE = -sin(theta4).*(L2Y_s.*cos(theta1+theta2)+L1Y_s.*cos(theta1)+L3Y_s.*cos(theta1+theta2+theta3));
if nargout > 1
    YE = cos(theta4).*(L2Y_s.*cos(theta1+theta2)+L1Y_s.*cos(theta1)+L3Y_s.*cos(theta1+theta2+theta3));
end
if nargout > 2
    ZE = L2Y_s.*sin(theta1+theta2)+L1Y_s.*sin(theta1)+L3Y_s.*sin(theta1+theta2+theta3);
end

== matlab function bhxxx_SL/Create_PLANT_BUS/CALC_BUS/THE_A_EFF_and_O_and_G ==
  data: L1Y_s input; AF_pos_eff output; L2Y_s input; L3Y_s input; theta1 input; theta2 input; theta3 input; AF_pos_O1 output; AF_pos_O2 output; AF_pos_O3 output; AF_pos_G1 output; AF_pos_G2 output; AF_pos_G3 output
function [AF_pos_eff,AF_pos_O1,AF_pos_O2,AF_pos_O3,AF_pos_G1,AF_pos_G2,AF_pos_G3] = THE_A_EFF_and_O_and_G(L1Y_s,L2Y_s,L3Y_s,theta1,theta2,theta3)
%#codegen

%    This function was generated by the Symbolic Math Toolbox version 7.0.
%    15-Sep-2016 15:54:05

AF_pos_eff = [0.0;L2Y_s.*cos(theta1+theta2)+L1Y_s.*cos(theta1)+L3Y_s.*cos(theta1+theta2+theta3);L2Y_s.*sin(theta1+theta2)+L1Y_s.*sin(theta1)+L3Y_s.*sin(theta1+theta2+theta3)];
if nargout > 1
    AF_pos_O1 = [0.0;0.0;0.0];
end
if nargout > 2
    AF_pos_O2 = [0.0;L1Y_s.*cos(theta1);L1Y_s.*sin(theta1)];
end
if nargout > 3
    AF_pos_O3 = [0.0;L2Y_s.*cos(theta1+theta2)+L1Y_s.*cos(theta1);L2Y_s.*sin(theta1+theta2)+L1Y_s.*sin(theta1)];
end
if nargout > 4
    AF_pos_G1 = [0.0;L1Y_s.*cos(theta1).*(1.0./2.0);L1Y_s.*sin(theta1).*(1.0./2.0)];
end
if nargout > 5
    AF_pos_G2 = [0.0;L2Y_s.*cos(theta1+theta2).*(1.0./2.0)+L1Y_s.*cos(theta1);L2Y_s.*sin(theta1+theta2).*(1.0./2.0)+L1Y_s.*sin(theta1)];
end
if nargout > 6
    AF_pos_G3 = [0.0;L2Y_s.*cos(theta1+theta2)+L1Y_s.*cos(theta1)+L3Y_s.*cos(theta1+theta2+theta3).*(1.0./2.0);L2Y_s.*sin(theta1+theta2)+L1Y_s.*sin(theta1)+L3Y_s.*sin(theta1+theta2+theta3).*(1.0./2.0)];
end

== matlab function bhxxx_SL/Create_PLANT_BUS/CALC_BUS/THE_W_EFF_and_O_and_G ==
  data: L1Y_s input; WF_pos_eff output; L2Y_s input; L3Y_s input; theta1 input; theta2 input; theta3 input; theta4 input; WF_pos_O1 output; WF_pos_O2 output; WF_pos_O3 output; WF_pos_G1 output; WF_pos_G2 output; WF_pos_G3 output
function [WF_pos_eff,WF_pos_O1,WF_pos_O2,WF_pos_O3,WF_pos_G1,WF_pos_G2,WF_pos_G3] = THE_W_EFF_and_O_and_G(L1Y_s,L2Y_s,L3Y_s,theta1,theta2,theta3,theta4)
%#codegen

%    This function was generated by the Symbolic Math Toolbox version 7.0.
%    15-Sep-2016 15:32:27

WF_pos_eff = [-sin(theta4).*(L2Y_s.*cos(theta1+theta2)+L1Y_s.*cos(theta1)+L3Y_s.*cos(theta1+theta2+theta3));cos(theta4).*(L2Y_s.*cos(theta1+theta2)+L1Y_s.*cos(theta1)+L3Y_s.*cos(theta1+theta2+theta3));L2Y_s.*sin(theta1+theta2)+L1Y_s.*sin(theta1)+L3Y_s.*sin(theta1+theta2+theta3)];
if nargout > 1
    WF_pos_O1 = [0.0;0.0;0.0];
end
if nargout > 2
    WF_pos_O2 = [-L1Y_s.*cos(theta1).*sin(theta4);L1Y_s.*cos(theta1).*cos(theta4);L1Y_s.*sin(theta1)];
end
if nargout > 3
    WF_pos_O3 = [-sin(theta4).*(L2Y_s.*cos(theta1+theta2)+L1Y_s.*cos(theta1));cos(theta4).*(L2Y_s.*cos(theta1+theta2)+L1Y_s.*cos(theta1));L2Y_s.*sin(theta1+theta2)+L1Y_s.*sin(theta1)];
end
if nargout > 4
    WF_pos_G1 = [L1Y_s.*cos(theta1).*sin(theta4).*(-1.0./2.0);L1Y_s.*cos(theta1).*cos(theta4).*(1.0./2.0);L1Y_s.*sin(theta1).*(1.0./2.0)];
end
if nargout > 5
    WF_pos_G2 = [-sin(theta4).*(L2Y_s.*cos(theta1+theta2).*(1.0./2.0)+L1Y_s.*cos(theta1));cos(theta4).*(L2Y_s.*cos(theta1+theta2).*(1.0./2.0)+L1Y_s.*cos(theta1));L2Y_s.*sin(theta1+theta2).*(1.0./2.0)+L1Y_s.*sin(theta1)];
end
if nargout > 6
    WF_pos_G3 = [-sin(theta4).*(L2Y_s.*cos(theta1+theta2)+L1Y_s.*cos(theta1)+L3Y_s.*cos(theta1+theta2+theta3).*(1.0./2.0));cos(theta4).*(L2Y_s.*cos(theta1+theta2)+L1Y_s.*cos(theta1)+L3Y_s.*cos(theta1+theta2+theta3).*(1.0./2.0));L2Y_s.*sin(theta1+theta2)+L1Y_s.*sin(theta1)+L3Y_s.*sin(theta1+theta2+theta3).*(1.0./2.0)];
end

== matlab function bhxxx_SL/Create_PLANT_BUS/Subsystem1/MATLAB Function ==
  data: r input size=[3 1]; TQ output; F input size=[3 1]
function TQ = CROSS(r,F)
%#codegen

TQ = cross(r,F);

== matlab function bhxxx_SL/Create_PLANT_BUS/Subsystem1/MATLAB Function1 ==
  data: r input size=[3 1]; TQ output; F input size=[3 1]
function TQ = CROSS(r,F)
%#codegen

TQ = cross(r,F);

== matlab function bhxxx_SL/Create_PLANT_BUS/Subsystem1/MATLAB Function2 ==
  data: r input size=[3 1]; TQ output; F input size=[3 1]
function TQ = CROSS(r,F)
%#codegen

TQ = cross(r,F);

== matlab function bhxxx_SL/Create_PLANT_BUS/Subsystem1/MATLAB Function3 ==
  data: r input size=[3 1]; TQ output; F input size=[3 1]
function TQ = CROSS(r,F)
%#codegen

TQ = cross(r,F);

== matlab function bhxxx_SL/Create_PLANT_BUS/Subsystem1/MATLAB Function4 ==
  data: r input size=[3 1]; TQ output; F input size=[3 1]
function TQ = CROSS(r,F)
%#codegen

TQ = cross(r,F);

== matlab function bhxxx_SL/Create_PLANT_BUS/Subsystem1/MATLAB Function5 ==
  data: r input size=[3 1]; TQ output; F input size=[3 1]
function TQ = CROSS(r,F)
%#codegen

TQ = cross(r,F);
